simulink model "collect_staic_data"  (R2023b)
settings: Solver=FixedStepDiscrete  StartTime=0.0  StopTime=10.0  FixedStep=5e-5  RelTol=1e-3
PreLoadFcn:
  | Simulink.defineIntEnumType('windowCommand', {'Off','Speed1','Speed2','Speed3'},[0,1,2,3])
libraries: simulink x1
settings Model: Creator=kz1nz0  LastModifiedBy=Ja

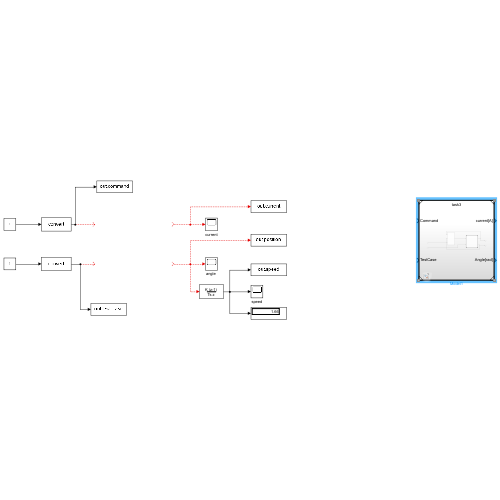
[thumbnail: Simulink's stored preview of the top-level diagram]
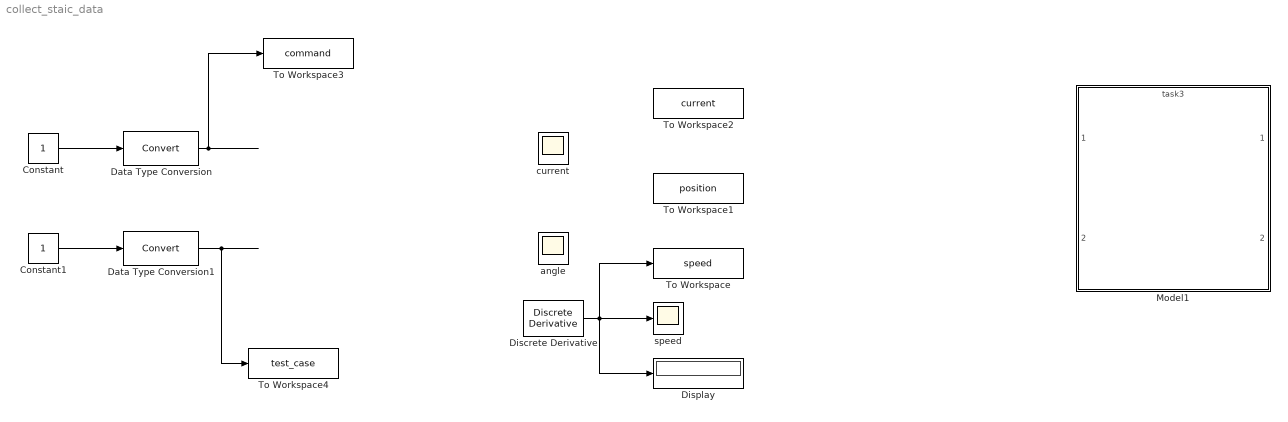
== system collect_staic_data ==
  Constant : Constant  OutDataTypeStr=int32
  Constant1 : Constant
  Data Type Conversion : DataTypeConversion  SaturateOnIntegerOverflow=off  RndMeth=Floor
  Data Type Conversion1 : DataTypeConversion  SaturateOnIntegerOverflow=off  RndMeth=Floor
  Discrete Derivative : simulink/Discrete/Discrete Derivative  gainval=1.0  ICPrevScaledInput=0.0  OutMin=[]  OutMax=[]  OutDataType=fixdt(1, 16)  OutScaling=2^-10  DoSatur=off
  Display : Display
  Model1 : ModelReference  ModelNameDialog=task3.slx  SimulationMode=Normal  ModelReferenceVersion=1.11
  To Workspace : ToWorkspace  VariableName=speed  SaveFormat=Timeseries  SampleTime=-1
  To Workspace1 : ToWorkspace  VariableName=position  SaveFormat=Timeseries  SampleTime=-1
  To Workspace2 : ToWorkspace  VariableName=current  SaveFormat=Timeseries  SampleTime=-1
  To Workspace3 : ToWorkspace  VariableName=command  SaveFormat=Timeseries  SampleTime=-1
  To Workspace4 : ToWorkspace  VariableName=test_case  SaveFormat=Timeseries  SampleTime=-1
  "angle " : Scope
  current : Scope
  speed : Scope
  wires:
  Constant/1 -> Data Type Conversion/1
  Constant1/1 -> Data Type Conversion1/1
  ? -> To Workspace2/1, current/1
  ? -> Discrete Derivative/1, To Workspace1/1, "angle "/1
  Data Type Conversion/1 -> To Workspace3/1
  Data Type Conversion1/1 -> To Workspace4/1
  Discrete Derivative/1 -> To Workspace/1, speed/1, Display/1
